simulink model "CO2_Insufflator"  (R2024b)
settings: Solver=VariableStepAuto  StartTime=0.0  StopTime=250  RelTol=1e-3
libraries: fl_lib x23, nesl_utility x9, SimscapeFluids_lib x6, slpidlib x2
(part 3 of 3)

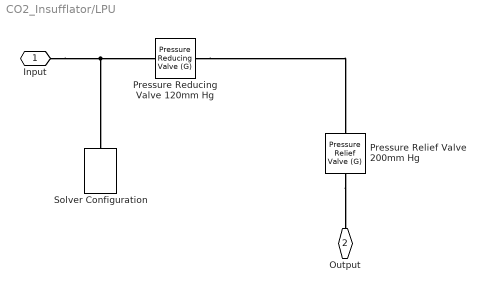
== system CO2_Insufflator/LPU ==
  Pressure Reducing Valve 120mm Hg : SimscapeFluids_lib/Gas/Valves & Orifices/Pressure Control Valves/Pressure Reducing Valve (G)  valve_parameterization=fluids.gas.valves_orifices.enum.OrificeParameterization.Cv  opening_characteristic=fluids.gas.valves_orifices.enum.OpeningCharacteristics.Linear  p_set_gauge=0.16 bar  p_range=0.1 bar  Cv_max=4  p_gauge_Cv_TLU=0.2 : 0.2 : 1.2 MPa  Cv_TLU=[4, 3.2, 2.4, 1.6, .8, 1e-06]  xT_Cv=0.7  Kv_max=3.6  p_gauge_Kv_TLU=0.2 : 0.2 : 1.2 MPa  Kv_TLU=[3.6, 2.88, 2.16, 1.44, .72, 1e-06]  xT_Kv=0.7  C_max=12 l/(bar*s)  B_crit_linear=0.3  p_gauge_C_TLU=0.2 : 0.2 : 1.2 MPa  C_TLU=[12, 9.6, 7.2, 4.8, 2.4, 1e-05] l/(bar*s)  B_crit_TLU=0.3 * ones(1, 6)  m=0.5  T_ref_C=293.15 K  rho_ref_C=1.185 kg/m^3  orifice_area_max=1e-4 m^2  p_gauge_orifice_area_TLU=0.2 : 0.2 : 1.2 MPa  orifice_area_TLU=[.0001, 8e-05, 6e-05, 4e-05, 2e-05, 1e-10] m^2  Cd=0.64  leakage_fraction=1e-6  smoothing_factor=0.01  B_lam=0.999  area=0.01 m^2
      settings: InternalSimscapePortConfiguration="{\"Bottom\":[],\"Left\":[{\"id\":\"A\",\"label\":\"A\",\"type\":\"foundation.gas.gas\"}],\"Right\":[{\"id\":\"B\",\"label\":\"B\",\"type\":\"foundation.gas.gas\"}],\"Top\":[]}"
  Pressure Relief Valve 200mm Hg : SimscapeFluids_lib/Gas/Valves & Orifices/Pressure Control Valves/Pressure Relief Valve (G)  opening_pressure_spec=fluids.gas.valves_orifices.enum.PressureControlSpec.PressureDifference  valve_parameterization=fluids.gas.valves_orifices.enum.OrificeParameterization.Cv  opening_characteristic=fluids.gas.valves_orifices.enum.OpeningCharacteristics.Linear  p_set_differential=0.26 bar  p_set_gauge=0.1 MPa  p_range=0.1 bar  Cv_max=4  p_diff_Cv_TLU=0.2 : 0.2 : 1.2 MPa  p_gauge_Cv_TLU=0.2 : 0.2 : 1.2 MPa  Cv_TLU=[1e-06, .8, 1.6, 2.4, 3.2, 4]  xT_Cv=0.7  Kv_max=3.6  p_diff_Kv_TLU=0.2 : 0.2 : 1.2 MPa  p_gauge_Kv_TLU=0.2 : 0.2 : 1.2 MPa  Kv_TLU=[1e-06, .72, 1.44, 2.16, 2.88, 3.6]  xT_Kv=0.7  C_max=12 l/(bar*s)  B_crit_linear=0.3  p_diff_C_TLU=0.2 : 0.2 : 1.2 MPa  p_gauge_C_TLU=0.2 : 0.2 : 1.2 MPa  C_TLU=[1e-05, 2.4, 4.8, 7.2, 9.6, 12] l/(bar*s)  B_crit_TLU=0.3 * ones(1, 6)  m=0.5  T_ref_C=293.15 K  rho_ref_C=1.185 kg/m^3  orifice_area_max=1e-4 m^2  p_diff_orifice_area_TLU=0.2 : 0.2 : 1.2 MPa  p_gauge_orifice_area_TLU=0.2 : 0.2 : 1.2 MPa  orifice_area_TLU=[1e-10, 2e-05, 4e-05, 6e-05, 8e-05, .0001] m^2  Cd=0.64  leakage_fraction=1e-6  smoothing_factor=0.01  B_lam=0.999  area=0.01 m^2
      settings: InternalSimscapePortConfiguration="{\"Bottom\":[],\"Left\":[{\"id\":\"A\",\"label\":\"A\",\"type\":\"foundation.gas.gas\"}],\"Right\":[{\"id\":\"B\",\"label\":\"B\",\"type\":\"foundation.gas.gas\"}],\"Top\":[]}"
  Solver Configuration : nesl_utility/Solver Configuration  PhysicalDomain=network_engine_domain  SubClassName=solver  LeftPortType=input  RightPortType=generic  Tones=[]  Harmonics=[]  SimulateNoise=off  Profile=off  UseLocalSampling=off  EnableSwitchedLinearOptims=on  FrequencyDomain=off  UseCCode=off  RelTol=0.001  AbsTol=0.001  MinStep=1e-09  ToWorkspace=off  RevertToSquareIcSolve=off  NumHomotopyIterations=100  PhasorMode=off  PhasorModeNumHarmonics=1  ConsistencySolver=NEWTON_XTOL_AFTER_FTOL  IndexReductionMethod=DerivativeReplacement  DoDC=off  ResidualTolerance=1e-09  ConsistencyTolSource=GLOBAL  ConsistencyAbsTol=0.001  ConsistencyRelTol=0.001  ConsistencyTolFactor=0.001  UseLocalSolver=off  LocalSolverChoice=NE_BACKWARD_EULER_ADVANCER  ResolveIndetEquations=on  FunctionEvalNumThread=1  LocalSolverSampleTime=0.001  DoFixedCost=off  MaxNonlinIter=3  MaxModeIter=2  ComputeImpulses=off  ImpulseIterations=2  LinearAlgebra=auto  LinearAlgebraNumThread=0  EquationFormulation=NE_TIME_EF  DelaysMemoryBudget=1024  AutomaticFiltering=on  FilteringTimeConstant=0.001  PartitionStorageMethod=AS_NEEDED  PartitionMemoryBudget=1024  PartitionMethod=ROBUST  MultibodyUseLocalSolver=off  MultibodyLocalSolverChoice=ODE1  MultibodyLocalSolverSampleTime=0.001
  Input : PMIOPort  Side=Left
  Output : PMIOPort  Port=2  Side=Right
  connections:
  Pressure Relief Valve 200mm Hg/RConn1 -- Output/RConn1
  Pressure Reducing Valve 120mm Hg/RConn1 -- Pressure Relief Valve 200mm Hg/LConn1
  Input/RConn1 -- Solver Configuration/RConn1 -- Pressure Reducing Valve 120mm Hg/LConn1

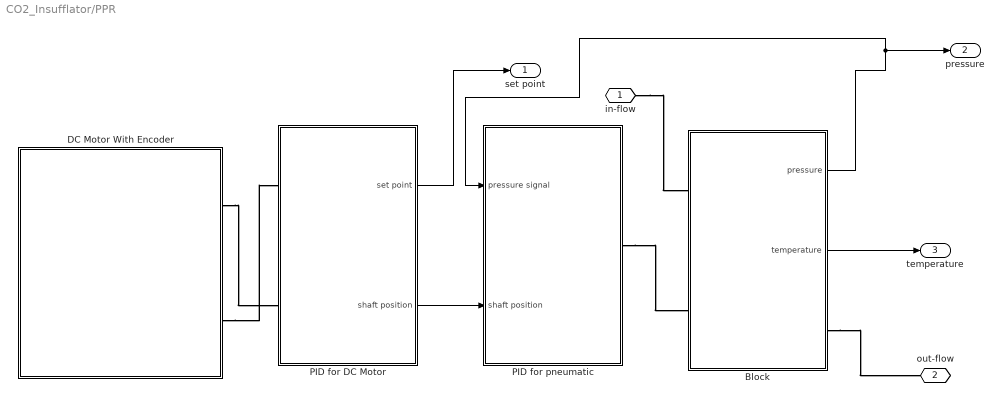
== system CO2_Insufflator/PPR ==
  Block : Subsystem
  DC Motor With Encoder : Subsystem
  PID for DC Motor : Subsystem
  PID for pneumatic : Subsystem
  in-flow : PMIOPort  Side=Left
  out-flow : PMIOPort  Port=2  Side=Left
  set point : Outport
  pressure : Outport  Port=2
  temperature : Outport  Port=3
  wires:
  PID for DC Motor/1(set point) -> set point/1
  Block/1(pressure) -> PID for pneumatic/1(pressure signal), pressure/1
  Block/2(temperature) -> temperature/1
  PID for DC Motor/2(shaft position) -> PID for pneumatic/2(shaft position)
  connections:
  DC Motor With Encoder/LConn1 -- PID for DC Motor/LConn2
  DC Motor With Encoder/LConn2 -- PID for DC Motor/LConn1
  in-flow/RConn1 -- Block/LConn1
  Block/RConn1 -- out-flow/RConn1
  PID for pneumatic/RConn1 -- Block/LConn2

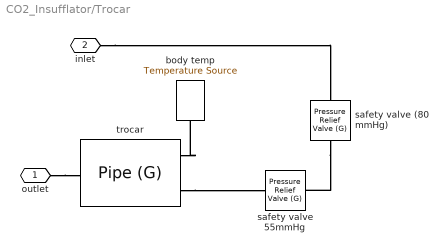
== system CO2_Insufflator/Trocar ==
  body temp : fl_lib/Thermal/Thermal Sources/Temperature Source  temperature=37 degC
  safety valve (80 mmHg) : SimscapeFluids_lib/Gas/Valves & Orifices/Pressure Control Valves/Pressure Relief Valve (G)  opening_pressure_spec=fluids.gas.valves_orifices.enum.PressureControlSpec.PressureDifference  valve_parameterization=fluids.gas.valves_orifices.enum.OrificeParameterization.Cv  opening_characteristic=fluids.gas.valves_orifices.enum.OpeningCharacteristics.Linear  p_set_differential=0.1053 bar  p_set_gauge=0.1 MPa  p_range=0.1 MPa  Cv_max=4  p_diff_Cv_TLU=0.2 : 0.2 : 1.2 MPa  p_gauge_Cv_TLU=0.2 : 0.2 : 1.2 MPa  Cv_TLU=[1e-06, .8, 1.6, 2.4, 3.2, 4]  xT_Cv=0.7  Kv_max=3.6  p_diff_Kv_TLU=0.2 : 0.2 : 1.2 MPa  p_gauge_Kv_TLU=0.2 : 0.2 : 1.2 MPa  Kv_TLU=[1e-06, .72, 1.44, 2.16, 2.88, 3.6]  xT_Kv=0.7  C_max=12 l/(bar*s)  B_crit_linear=0.3  p_diff_C_TLU=0.2 : 0.2 : 1.2 MPa  p_gauge_C_TLU=0.2 : 0.2 : 1.2 MPa  C_TLU=[1e-05, 2.4, 4.8, 7.2, 9.6, 12] l/(bar*s)  B_crit_TLU=0.3 * ones(1, 6)  m=0.5  T_ref_C=293.15 K  rho_ref_C=1.185 kg/m^3  orifice_area_max=1e-4 m^2  p_diff_orifice_area_TLU=0.2 : 0.2 : 1.2 MPa  p_gauge_orifice_area_TLU=0.2 : 0.2 : 1.2 MPa  orifice_area_TLU=[1e-10, 2e-05, 4e-05, 6e-05, 8e-05, .0001] m^2  Cd=0.64  leakage_fraction=1e-6  smoothing_factor=0.01  B_lam=0.999  area=0.01 m^2
      settings: InternalSimscapePortConfiguration="{\"Bottom\":[],\"Left\":[{\"id\":\"A\",\"label\":\"A\",\"type\":\"foundation.gas.gas\"}],\"Right\":[{\"id\":\"B\",\"label\":\"B\",\"type\":\"foundation.gas.gas\"}],\"Top\":[]}"
  safety valve 55mmHg : SimscapeFluids_lib/Gas/Valves & Orifices/Pressure Control Valves/Pressure Relief Valve (G)  opening_pressure_spec=fluids.gas.valves_orifices.enum.PressureControlSpec.PressureDifference  valve_parameterization=fluids.gas.valves_orifices.enum.OrificeParameterization.Cv  opening_characteristic=fluids.gas.valves_orifices.enum.OpeningCharacteristics.Linear  p_set_differential=0.0724 bar  p_set_gauge=0.1 MPa  p_range=0.1 MPa  Cv_max=4  p_diff_Cv_TLU=0.2 : 0.2 : 1.2 MPa  p_gauge_Cv_TLU=0.2 : 0.2 : 1.2 MPa  Cv_TLU=[1e-06, .8, 1.6, 2.4, 3.2, 4]  xT_Cv=0.7  Kv_max=3.6  p_diff_Kv_TLU=0.2 : 0.2 : 1.2 MPa  p_gauge_Kv_TLU=0.2 : 0.2 : 1.2 MPa  Kv_TLU=[1e-06, .72, 1.44, 2.16, 2.88, 3.6]  xT_Kv=0.7  C_max=12 l/(bar*s)  B_crit_linear=0.3  p_diff_C_TLU=0.2 : 0.2 : 1.2 MPa  p_gauge_C_TLU=0.2 : 0.2 : 1.2 MPa  C_TLU=[1e-05, 2.4, 4.8, 7.2, 9.6, 12] l/(bar*s)  B_crit_TLU=0.3 * ones(1, 6)  m=0.5  T_ref_C=293.15 K  rho_ref_C=1.185 kg/m^3  orifice_area_max=1e-4 m^2  p_diff_orifice_area_TLU=0.2 : 0.2 : 1.2 MPa  p_gauge_orifice_area_TLU=0.2 : 0.2 : 1.2 MPa  orifice_area_TLU=[1e-10, 2e-05, 4e-05, 6e-05, 8e-05, .0001] m^2  Cd=0.64  leakage_fraction=1e-6  smoothing_factor=0.01  B_lam=0.999  area=0.01 m^2
      settings: InternalSimscapePortConfiguration="{\"Bottom\":[],\"Left\":[{\"id\":\"A\",\"label\":\"A\",\"type\":\"foundation.gas.gas\"}],\"Right\":[{\"id\":\"B\",\"label\":\"B\",\"type\":\"foundation.gas.gas\"}],\"Top\":[]}"
  trocar : fl_lib/Gas/Elements/Pipe (G)  length=5 m  area=0.01 m^2  Dh=0.1 m  length_add=0.1 m  roughness=15e-6 m  Re_lam=2000  Re_tur=4000  shape_factor=64  Nu_lam=3.66  p_I_specify=off  p_I_priority=High  p_I=0.101325 MPa  p_I_nominal_specify=off  p_I_nominal_value=1  p_I_nominal_unit=MPa  T_I_specify=off  T_I_priority=High  T_I=293.15 K  T_I_nominal_specify=off  T_I_nominal_value=1  T_I_nominal_unit=K  rho_I_specify=off  rho_I_priority=None  rho_I=1.2 kg/m^3  rho_I_nominal_specify=off  rho_I_nominal_value=1  rho_I_nominal_unit=kg/m^3
  outlet : PMIOPort  Side=Left
  inlet : PMIOPort  Port=2  Side=Right
  connections:
  inlet/RConn1 -- safety valve (80 mmHg)/LConn1
  safety valve (80 mmHg)/RConn1 -- safety valve 55mmHg/LConn1
  trocar/LConn1 -- safety valve 55mmHg/RConn1
  outlet/RConn1 -- trocar/RConn1
  trocar/LConn2 -- body temp/LConn1

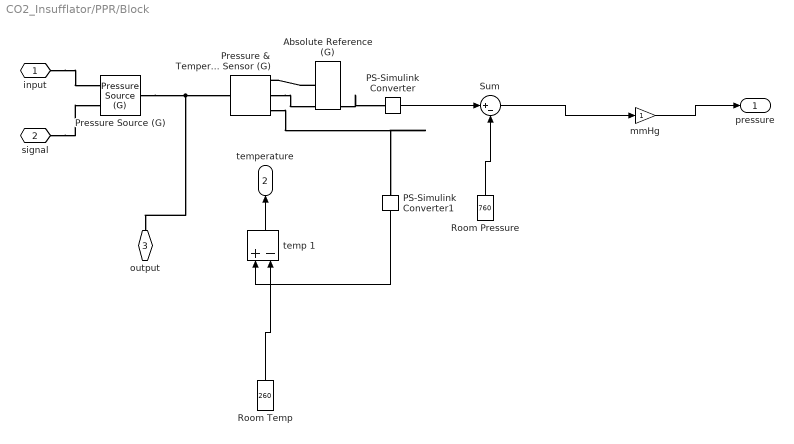
== system CO2_Insufflator/PPR/Block ==
  Absolute Reference (G) : fl_lib/Gas/Elements/Absolute Reference (G)
      settings: InternalSimscapePortConfiguration="{\"Bottom\":[],\"Left\":[{\"id\":\"A\",\"label\":\"\",\"type\":\"foundation.gas.gas\"}],\"Right\":[],\"Top\":[]}"
  PS-Simulink Converter : nesl_utility/PS-Simulink Converter  PhysicalDomain=network_engine_domain  SubClassName=ps_output  LeftPortType=input  RightPortType=output  PseudoPeriodic=off  Frequencies=[]  VectorFormat=inherit  Unit=inherit  AffineConversion=off
  PS-Simulink Converter1 : nesl_utility/PS-Simulink Converter  PhysicalDomain=network_engine_domain  SubClassName=ps_output  LeftPortType=input  RightPortType=output  PseudoPeriodic=off  Frequencies=[]  VectorFormat=inherit  Unit=inherit  AffineConversion=off
  Pressure & Temperature Sensor (G) : fl_lib/Gas/Sensors/Pressure & Temperature Sensor (G)  reference=foundation.enum.MeasurementReference.difference  pressure=true  pressure_spec=foundation.enum.PressureMeasementSpec.Absolute  temperature=true
      settings: InternalSimscapePortConfiguration="{\"Bottom\":[{\"id\":\"T\",\"label\":\"T\",\"type\":\"output\"}],\"Left\":[{\"id\":\"A\",\"label\":\"A\",\"type\":\"foundation.gas.gas\"}],\"Right\":[{\"id\":\"B\",\"label\":\"B\",\"type\":\"foundation.gas.gas\"},{\"id\":\"P\",\"label\":\"P\",\"type\":\"output\"}],\"Top\":[]}"
  Pressure Source (G) : fl_lib/Gas/Sources/Pressure Source (G)  source_type=foundation.enum.constant_controlled.controlled  pressure_differential=0 MPa  power_spec=foundation.enum.power_spec.isentropic  area_A=0.01 m^2  area_B=0.01 m^2
      settings: InternalSimscapePortConfiguration="{\"Bottom\":[],\"Left\":[{\"id\":\"A\",\"label\":\"A\",\"type\":\"foundation.gas.gas\"},{\"id\":\"P\",\"label\":\"P\",\"type\":\"input\"}],\"Right\":[{\"id\":\"B\",\"label\":\"B\",\"type\":\"foundation.gas.gas\"}],\"Top\":[]}"
  Room Pressure : Constant  Value=760
  Room Temp : Constant  Value=260
  Sum : Sum  Inputs=|+-
  mmHg : Gain
  temp 1 : Sum  Inputs=+-
  input : PMIOPort  Side=Left
  signal : PMIOPort  Port=2  Side=Left
  output : PMIOPort  Port=3  Side=Right
  pressure : Outport
  temperature : Outport  Port=2
  wires:
  temp 1/1 -> temperature/1
  mmHg/1 -> pressure/1
  Sum/1 -> mmHg/1
  PS-Simulink Converter/1 -> Sum/1
  Room Pressure/1 -> Sum/2
  Room Temp/1 -> temp 1/2
  PS-Simulink Converter1/1 -> temp 1/1
  connections:
  input/RConn1 -- Pressure Source (G)/LConn1
  signal/RConn1 -- Pressure Source (G)/LConn2
  Pressure Source (G)/RConn1 -- output/RConn1 -- Pressure & Temperature Sensor (G)/LConn1
  Pressure & Temperature Sensor (G)/RConn2 -- PS-Simulink Converter/LConn1
  Absolute Reference (G)/LConn1 -- Pressure & Temperature Sensor (G)/RConn1
  Pressure & Temperature Sensor (G)/RConn3 -- PS-Simulink Converter1/LConn1

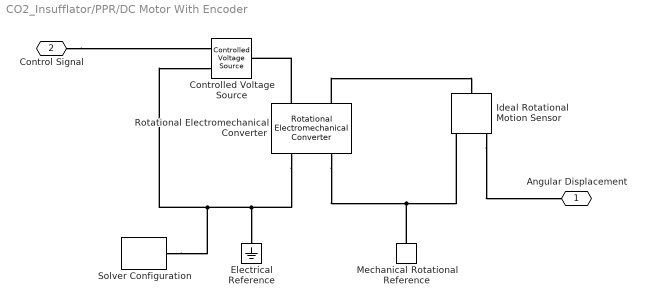
== system CO2_Insufflator/PPR/DC Motor With Encoder ==
  Controlled Voltage Source : fl_lib/Electrical/Electrical Sources/Controlled Voltage Source
  Electrical Reference : fl_lib/Electrical/Electrical Elements/Electrical Reference
  Ideal Rotational Motion Sensor : fl_lib/Mechanical/Mechanical Sensors/Ideal Rotational Motion Sensor  reference=foundation.enum.MeasurementReference.difference  acceleration_port=false  velocity_port=true  position_port=true  wrap_angle=false  offset=0 rad
  Mechanical Rotational Reference : fl_lib/Mechanical/Rotational Elements/Mechanical Rotational Reference
  Rotational Electromechanical Converter : fl_lib/Electrical/Electrical Elements/Rotational Electromechanical Converter  K=0.1 V*s/rad  i_specify=off  i_priority=None  i=0 A  i_nominal_specify=off  i_nominal_value=1  i_nominal_unit=A  v_specify=off  v_priority=None  v=0 V  v_nominal_specify=off  v_nominal_value=1  v_nominal_unit=V  t_specify=off  t_priority=None  t=0 N*m  t_nominal_specify=off  t_nominal_value=1  t_nominal_unit=N*m  w_specify=off  w_priority=None  w=0 rad/s  w_nominal_specify=off  w_nominal_value=1  w_nominal_unit=rad/s
  Solver Configuration : nesl_utility/Solver Configuration  PhysicalDomain=network_engine_domain  SubClassName=solver  LeftPortType=input  RightPortType=generic  Tones=[]  Harmonics=[]  SimulateNoise=off  Profile=off  UseLocalSampling=off  EnableSwitchedLinearOptims=on  FrequencyDomain=off  UseCCode=off  RelTol=0.001  AbsTol=0.001  MinStep=1e-09  ToWorkspace=off  RevertToSquareIcSolve=off  NumHomotopyIterations=100  PhasorMode=off  PhasorModeNumHarmonics=1  ConsistencySolver=NEWTON_XTOL_AFTER_FTOL  IndexReductionMethod=DerivativeReplacement  DoDC=off  ResidualTolerance=1e-09  ConsistencyTolSource=GLOBAL  ConsistencyAbsTol=0.001  ConsistencyRelTol=0.001  ConsistencyTolFactor=0.001  UseLocalSolver=off  LocalSolverChoice=NE_BACKWARD_EULER_ADVANCER  ResolveIndetEquations=on  FunctionEvalNumThread=1  LocalSolverSampleTime=0.001  DoFixedCost=off  MaxNonlinIter=3  MaxModeIter=2  ComputeImpulses=off  ImpulseIterations=2  LinearAlgebra=auto  LinearAlgebraNumThread=0  EquationFormulation=NE_TIME_EF  DelaysMemoryBudget=1024  AutomaticFiltering=on  FilteringTimeConstant=0.001  PartitionStorageMethod=AS_NEEDED  PartitionMemoryBudget=1024  PartitionMethod=ROBUST  MultibodyUseLocalSolver=off  MultibodyLocalSolverChoice=ODE1  MultibodyLocalSolverSampleTime=0.001
  Angular Displacement : PMIOPort  Side=Left
  Control Signal : PMIOPort  Port=2  Side=Left
  connections:
  Control Signal/RConn1 -- Controlled Voltage Source/RConn1
  Ideal Rotational Motion Sensor/RConn3 -- Angular Displacement/RConn1
  Rotational Electromechanical Converter/LConn2 -- Ideal Rotational Motion Sensor/LConn1
  Rotational Electromechanical Converter/RConn2 -- Ideal Rotational Motion Sensor/RConn1 -- Mechanical Rotational Reference/LConn1
  Rotational Electromechanical Converter/LConn1 -- Controlled Voltage Source/LConn1
  Rotational Electromechanical Converter/RConn1 -- Electrical Reference/LConn1 -- Solver Configuration/RConn1 -- Controlled Voltage Source/RConn2

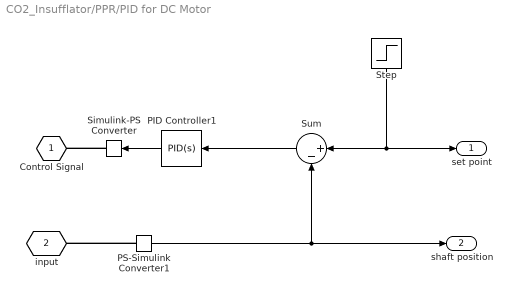
== system CO2_Insufflator/PPR/PID for DC Motor ==
  PID Controller1 : slpidlib/PID Controller  Controller=PID  Form=Parallel  TimeDomain=Continuous-time  UseExternalTs=off  SampleTime=-1  IntegratorMethod=Forward Euler  FilterMethod=Forward Euler  ControllerParametersSource=internal  P=1  I=1  UseKiTs=off  D=0  UseExternalDerivativeSource=off  N=100  UseFilter=on  TunerSelectOption=Transfer Function Based (PID Tuner App)  InitialConditionSource=internal  InitialConditionForIntegrator=0  InitialConditionForFilter=0  DifferentiatorICPrevScaledInput=0  ExternalReset=none  TrackingMode=off  Kt=1  LimitOutput=off  SatLimitsSource=internal  UpperSaturationLimit=inf  LowerSaturationLimit=-inf  LinearizeAsGain=on  AntiWindupMode=none  Kb=1  LimitIntegrator=off  UpperIntegratorSaturationLimit=inf  LowerIntegratorSaturationLimit=-inf  POutMin=[]  POutMax=[]  IOutMin=[]  IOutMax=[]  DOutMin=[]  DOutMax=[]  NOutMin=[]  NOutMax=[]  SumOutMin=[]  SumOutMax=[]  SaturationOutMin=[]  SaturationOutMax=[]  PParamMin=[]  PParamMax=[]  IParamMin=[]  IParamMax=[]  DParamMin=[]  DParamMax=[]  NParamMin=[]  NParamMax=[]  KbParamMin=[]  KbParamMax=[]  KtParamMin=[]  KtParamMax=[]  KbOutMin=[]  KbOutMax=[]  KtOutMin=[]  KtOutMax=[]  IntegratorOutMin=[]  IntegratorOutMax=[]  FilterOutMin=[]  FilterOutMax=[]  SumI1OutMin=[]  SumI1OutMax=[]  SumI2OutMin=[]  SumI2OutMax=[]  SumI3OutMin=[]  SumI3OutMax=[]  SumI4OutMin=[]  SumI4OutMax=[]  SumDOutMin=[]  SumDOutMax=[]  DifferentiatorOutMin=[]  DifferentiatorOutMax=[]  FilterDiffOutCoefMin=[]  FilterDiffOutCoefMax=[]  ReciprocalOutMin=[]  ReciprocalOutMax=[]  SumDenOutMin=[]  SumDenOutMax=[]  SumNumOutMin=[]  SumNumOutMax=[]  DivideOutMin=[]  DivideOutMax=[]  UdiffTsProdOutMin=[]  UdiffTsProdOutMax=[]  NTsProdOutMin=[]  NTsProdOutMax=[]  UintegralTsProdOutMin=[]  UintegralTsProdOutMax=[]  UngainTsProdOutMin=[]  UngainTsProdOutMax=[]  ClampingZeroOutDataTypeStr=Inherit: Inherit via back propagation  ClampingZeroOutMin=[]  ClampingZeroOutMax=[]  FilterDenConstantOutDataTypeStr=Inherit: Inherit via back propagation  FilterDenConstantOutMin=[]  FilterDenConstantOutMax=[]  PCopyOutDataTypeStr=Inherit: Inherit via back propagation  PCopyOutMin=[]  PCopyOutMax=[]  NCopyOutDataTypeStr=Inherit: Inherit via back propagation  NCopyOutMin=[]  NCopyOutMax=[]  IntegratorContinuousStateAttributes=''  IntegratorStateMustResolveToSignalObject=off  IntegratorRTWStateStorageClass=Auto  FilterContinuousStateAttributes=''  FilterStateMustResolveToSignalObject=off  FilterRTWStateStorageClass=Auto  ParallelPVariant=InternalParameters  IdealPVariant=Disabled  IVariant=InternalParameters  DVariant=InternalParameters  IntegratorVariant=Continuous  SatVariant=Disabled  AWVariant=Passthrough  PCopyVariant=Disabled  TRVariant=Disabled  FdbkBlocksVariant=Forward  IdealPFdbkVariant=Disabled  SatFdbkVariant=Disabled  DerivativeFilterVariant=ContFilter  NVariant=InternalParameters  NCopyVariant=Disabled  FilterICVariant=InternalICsFilter  IntegratorICVariant=InternalICs  ExternalResetVariant=Disabled  TRSumVariant=Passthrough  SumFdbkVariant=Disabled  SumVariant=Sum_PID  TsampFilterVariant=InternalTs  TsampNgainVariant=Passthrough  TsampIntegralVariant=Disabled_SignalSpec  ExternalSaturationOutDataTypeStr=Inherit: Same as second input  DerivativeSourceVariant=ErrorSignal  PreIntVariant=InternalPreInt
  PS-Simulink Converter1 : nesl_utility/PS-Simulink Converter  PhysicalDomain=network_engine_domain  SubClassName=ps_output  LeftPortType=input  RightPortType=output  PseudoPeriodic=off  Frequencies=[]  VectorFormat=inherit  Unit=inherit  AffineConversion=off
  Simulink-PS Converter : nesl_utility/Simulink-PS Converter  PhysicalDomain=network_engine_domain  SubClassName=ps_input  LeftPortType=input  RightPortType=output  PseudoPeriodic=off  Frequencies=[]  NoiseDistribution=none  NoiseParameters=[]  Unit=1  AffineConversion=off  FilteringAndDerivatives=provide  SimscapeFilterOrder=1  InputFilterTimeConstant=0.001  UdotUserProvided=0
  Step : Step  SampleTime=0
  Sum : Sum  Inputs=|+-
  Control Signal : PMIOPort  Side=Left
  input : PMIOPort  Port=2  Side=Left
  set point : Outport
  shaft position : Outport  Port=2
  wires:
  Sum/1 -> PID Controller1/1
  Step/1 -> set point/1, Sum/1
  PS-Simulink Converter1/1 -> shaft position/1, Sum/2
  PID Controller1/1 -> Simulink-PS Converter/1
  connections:
  PS-Simulink Converter1/LConn1 -- input/RConn1
  Simulink-PS Converter/RConn1 -- Control Signal/RConn1

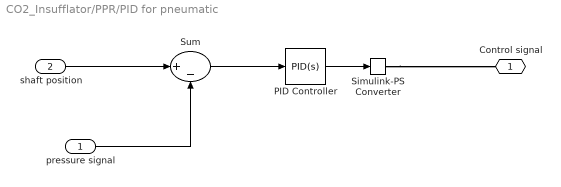
== system CO2_Insufflator/PPR/PID for pneumatic ==
  pressure signal : Inport
  shaft position : Inport  Port=2
  PID Controller : slpidlib/PID Controller  Controller=PID  Form=Parallel  TimeDomain=Continuous-time  UseExternalTs=off  SampleTime=-1  IntegratorMethod=Forward Euler  FilterMethod=Forward Euler  ControllerParametersSource=internal  P=1  I=1  UseKiTs=off  D=0  UseExternalDerivativeSource=off  N=100  UseFilter=on  TunerSelectOption=Transfer Function Based (PID Tuner App)  InitialConditionSource=internal  InitialConditionForIntegrator=0  InitialConditionForFilter=0  DifferentiatorICPrevScaledInput=0  ExternalReset=none  TrackingMode=off  Kt=1  LimitOutput=off  SatLimitsSource=internal  UpperSaturationLimit=inf  LowerSaturationLimit=-inf  LinearizeAsGain=on  AntiWindupMode=none  Kb=1  LimitIntegrator=off  UpperIntegratorSaturationLimit=inf  LowerIntegratorSaturationLimit=-inf  POutMin=[]  POutMax=[]  IOutMin=[]  IOutMax=[]  DOutMin=[]  DOutMax=[]  NOutMin=[]  NOutMax=[]  SumOutMin=[]  SumOutMax=[]  SaturationOutMin=[]  SaturationOutMax=[]  PParamMin=[]  PParamMax=[]  IParamMin=[]  IParamMax=[]  DParamMin=[]  DParamMax=[]  NParamMin=[]  NParamMax=[]  KbParamMin=[]  KbParamMax=[]  KtParamMin=[]  KtParamMax=[]  KbOutMin=[]  KbOutMax=[]  KtOutMin=[]  KtOutMax=[]  IntegratorOutMin=[]  IntegratorOutMax=[]  FilterOutMin=[]  FilterOutMax=[]  SumI1OutMin=[]  SumI1OutMax=[]  SumI2OutMin=[]  SumI2OutMax=[]  SumI3OutMin=[]  SumI3OutMax=[]  SumI4OutMin=[]  SumI4OutMax=[]  SumDOutMin=[]  SumDOutMax=[]  DifferentiatorOutMin=[]  DifferentiatorOutMax=[]  FilterDiffOutCoefMin=[]  FilterDiffOutCoefMax=[]  ReciprocalOutMin=[]  ReciprocalOutMax=[]  SumDenOutMin=[]  SumDenOutMax=[]  SumNumOutMin=[]  SumNumOutMax=[]  DivideOutMin=[]  DivideOutMax=[]  UdiffTsProdOutMin=[]  UdiffTsProdOutMax=[]  NTsProdOutMin=[]  NTsProdOutMax=[]  UintegralTsProdOutMin=[]  UintegralTsProdOutMax=[]  UngainTsProdOutMin=[]  UngainTsProdOutMax=[]  ClampingZeroOutDataTypeStr=Inherit: Inherit via back propagation  ClampingZeroOutMin=[]  ClampingZeroOutMax=[]  FilterDenConstantOutDataTypeStr=Inherit: Inherit via back propagation  FilterDenConstantOutMin=[]  FilterDenConstantOutMax=[]  PCopyOutDataTypeStr=Inherit: Inherit via back propagation  PCopyOutMin=[]  PCopyOutMax=[]  NCopyOutDataTypeStr=Inherit: Inherit via back propagation  NCopyOutMin=[]  NCopyOutMax=[]  IntegratorContinuousStateAttributes=''  IntegratorStateMustResolveToSignalObject=off  IntegratorRTWStateStorageClass=Auto  FilterContinuousStateAttributes=''  FilterStateMustResolveToSignalObject=off  FilterRTWStateStorageClass=Auto  ParallelPVariant=InternalParameters  IdealPVariant=Disabled  IVariant=InternalParameters  DVariant=InternalParameters  IntegratorVariant=Continuous  SatVariant=Disabled  AWVariant=Passthrough  PCopyVariant=Disabled  TRVariant=Disabled  FdbkBlocksVariant=Forward  IdealPFdbkVariant=Disabled  SatFdbkVariant=Disabled  DerivativeFilterVariant=ContFilter  NVariant=InternalParameters  NCopyVariant=Disabled  FilterICVariant=InternalICsFilter  IntegratorICVariant=InternalICs  ExternalResetVariant=Disabled  TRSumVariant=Passthrough  SumFdbkVariant=Disabled  SumVariant=Sum_PID  TsampFilterVariant=InternalTs  TsampNgainVariant=Passthrough  TsampIntegralVariant=Disabled_SignalSpec  ExternalSaturationOutDataTypeStr=Inherit: Same as second input  DerivativeSourceVariant=ErrorSignal  PreIntVariant=InternalPreInt
  Simulink-PS Converter : nesl_utility/Simulink-PS Converter  PhysicalDomain=network_engine_domain  SubClassName=ps_input  LeftPortType=input  RightPortType=output  PseudoPeriodic=off  Frequencies=[]  NoiseDistribution=none  NoiseParameters=[]  Unit=1  AffineConversion=off  FilteringAndDerivatives=provide  SimscapeFilterOrder=1  InputFilterTimeConstant=0.001  UdotUserProvided=0
  Sum : Sum  Inputs=|+-
  Control signal : PMIOPort  Side=Right
  wires:
  pressure signal/1 -> Sum/2
  shaft position/1 -> Sum/1
  Sum/1 -> PID Controller/1
  PID Controller/1 -> Simulink-PS Converter/1
  connections:
  Simulink-PS Converter/RConn1 -- Control signal/RConn1
